simulink model "lift_stateflow"  (R2024b)
settings: Solver=FixedStepAuto  StartTime=0.0  StopTime=250  FixedStep=1  RelTol=1e-3
settings Model: PacingRate=20  Creator=user  LastModifiedBy=user

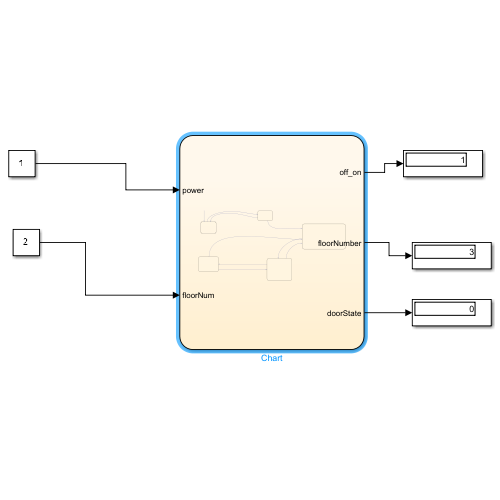
[thumbnail: Simulink's stored preview of the top-level diagram]
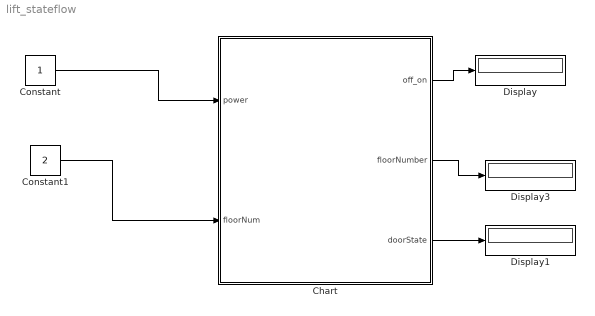
== system lift_stateflow ==
  Chart : Stateflow chart  TreatAsAtomicUnit=on
  Constant : Constant
  Constant1 : Constant  Value=2
  Display : Display
  Display1 : Display
  Display3 : Display
  wires:
  Constant/1 -> Chart/1(power)
  Constant1/1 -> Chart/2(floorNum)
  Chart/1(off_on) -> Display/1
  Chart/2(floorNumber) -> Display3/1
  Chart/3(doorState) -> Display1/1

== stateflow chart lift_stateflow/Chart ==
  settings: updateMethod=CONTINUOUS
  state status_on
    off_on=1;
  state status_off
    off_on=0;
  state floor_1
    entry:
    floorNumber=1;
    doorState=1;
    exit:
    doorState=0;
  state floor_3
    entry:
    floorNumber=3;
    doorState=1;
    exit:
    doorState=0;
  state floor_2
    entry:
    doorState=0;
    exit:
    doorState=0;
  (default) -> status_off
  status_off -> status_on : [power==1]
  status_on -> status_off [order 1] : [power==0]
  status_on -> floor_1 [order 2] : [floorNum==1 || floorNum==2 || floorNum==3]
  floor_3 -> floor_1 [order 1] : [floorNum==1&&after(30,sec)]
  floor_1 -> floor_2 : [floorNum==2||floorNum==3&&after(30,sec)]
  floor_2 -> floor_1 [order 2] : [floorNum==1&&after(30,sec)]
  floor_2 -> floor_3 [order 1] : [floorNum==3&&after(30,sec)]
  floor_3 -> floor_2 [order 2] : [floorNum==2&&after(30,sec)]
  data: off_on output; power input; floorNum input; floorNumber output; doorState output
